simulink model "ModeController"  (Simulink 7.6)
settings: Solver=ode45  StartTime=0.0  StopTime=10.0  RelTol=1e-3
settings Model: Creator=Zsolt  LastModifiedBy=bapty
settings HardwareCC: TargetIntDivRoundTo=Zero  TargetEndianess=LittleEndian  TargetHWDeviceType=MATLAB Host  ProdEqTarget=off
settings RTWCC: SystemTargetFile=rsim.tlc  TemplateMakefile=rsim_default_tmf  Description=Rapid Simulation Target  ProcessScript=rsim_make_rtw_hook
settings RSimTargetCC: TargetFunctionLibrary=ANSI_C  ERTMultiwordTypeDef=System defined  ERTCodeCoverageTool=None  ERTMultiwordLength=256  IsPILTarget=off  EnableShiftOperators=on  PortableWordSizes=off

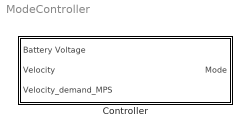
== system ModeController ==
  Controller : Subsystem

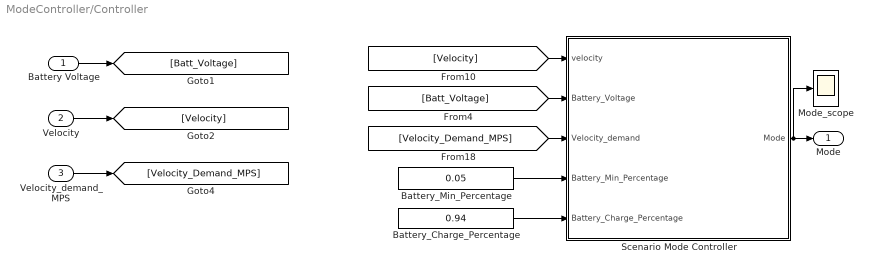
== system ModeController/Controller ==
  Battery Voltage : Inport
  Velocity : Inport  Port=2
  Velocity_demand_MPS : Inport  Port=3
  " Battery_Charge_Percentage" : Constant  Value=0.94
  Battery_Min_Percentage : Constant  Value=0.05
  Mode_scope : Scope
      settings: TimeRange=500  YMin=-1  YMax=3
  Scenario Mode Controller : Stateflow chart  TreatAsAtomicUnit=on
  Mode : Outport
  wires:
  " Battery_Charge_Percentage"/1 -> Scenario Mode Controller/5(Battery_Charge_Percentage)
  Battery_Min_Percentage/1 -> Scenario Mode Controller/4(Battery_Min_Percentage)
  Scenario Mode Controller/1(Mode) -> Mode_scope/1, Mode/1
  [Batt_Voltage] -> Scenario Mode Controller/2(Battery_Voltage)
  [Velocity] -> Scenario Mode Controller/1(velocity)
  [Velocity_Demand_MPS] -> Scenario Mode Controller/3(Velocity_demand)
  Battery Voltage/1 -> [Batt_Voltage]
  Velocity/1 -> [Velocity]
  Velocity_demand_MPS/1 -> [Velocity_Demand_MPS]

== matlab function Controller/Scenario Mode Controller ==
  data: velocity input double; Mode output double; Battery_Voltage input double; Velocity_demand input double; Battery_Min_Percentage input double; Battery_Charge_Percentage input double
function Mode  = fcn(velocity, Battery_Voltage, Velocity_demand, Battery_Min_Percentage, Battery_Charge_Percentage)
%#eml
if Battery_Voltage < 200*Battery_Min_Percentage
    Mode = 1; % DE ON, Battery charge
elseif velocity < Velocity_demand
    Mode = 0; % we need all energy   
elseif Battery_Voltage < 200*Battery_Charge_Percentage
    Mode = 1; % charge
else
    Mode = 2; % DE ON, Battery is disconnected
end

%Mode = 2; % DE ON, Battery is disconnected
